simulink model "flo1_2018a"  (R2018a)
settings: Solver=FixedStepAuto  StartTime=0.0  StopTime=inf  FixedStep=0.01  RelTol=1e-3  EnableMultiTasking=on
settings Model: EnablePacing=on  Creator=Florian  LastModifiedBy=Florian
settings SolverCC: AutoInsertRateTranBlk=on
settings DataIOCC: LimitDataPoints=on  ReturnWorkspaceOutputs=on
settings OptimizationCC: LifeSpan=inf
settings DebuggingCC: AllowSymbolicDim=off  SFUnexpectedBacktrackingDiag=warning  SFNoUnconditionalDefaultTransitionDiag=warning  SFExecutionAtInitializationDiag=none  SFMachineParentedDataDiag=error
settings CodeAppCC: StateflowObjectComments=on
settings GRTTargetCC: TargetLangStandard=C89/C90 (ANSI)
settings ConfigComp: CovMetricSettings=dw  CovSaveCumulativeToWorkspaceVar=on  CovSaveSingleToWorkspaceVar=on  CovExternalEMLEnable=off  CovSFcnEnable=off

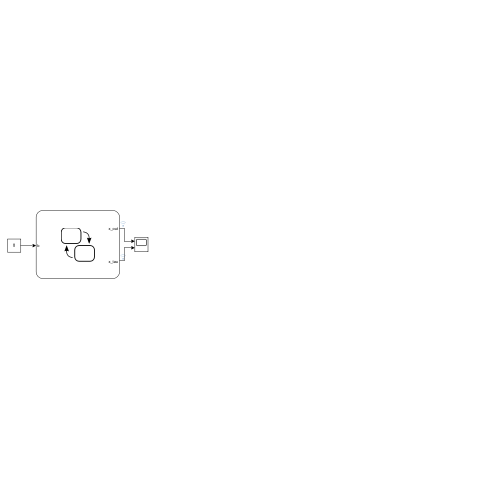
[thumbnail: Simulink's stored preview of the top-level diagram]
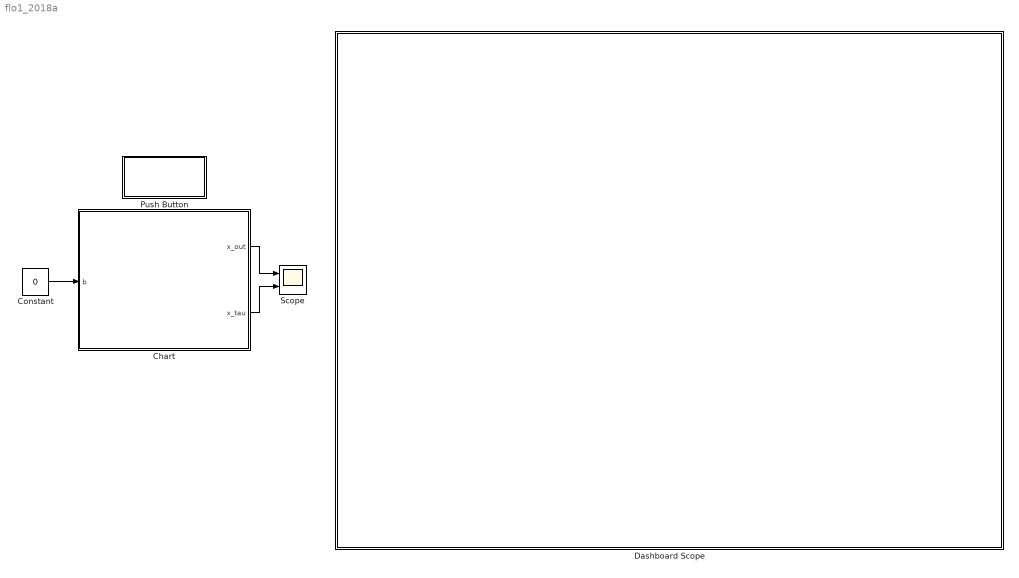
== system flo1_2018a ==
  Chart : Stateflow chart  TreatAsAtomicUnit=on
  Constant : Constant  Value=0
  Dashboard Scope : Subsystem  DialogController=hmiCreateDDGDialog  IsWebBlock=on  mask(MWDashboardBlock){webBlockId=8229a94b-91c7-4175-8aa9-2c0e1a5239d7, webBlockType=sdiscope, ShowInLibBrowser=on, ShowInitialText=on, HMISrcModelName=flo1_2018b}
      mask prompts: webBlockId "WebBlock Id"; webBlockType "WebBlock Type"; HMISrcModelName "Source Model"
      mask help: Traces signals on the dashboard scope during simulation.
      mask Help: helpview([docroot '/mapfiles/simulink.map'], 'hmi_scope')
      mask Display:
      | if strcmp(get_param(bdroot(gcb),'BlockDiagramType'),'library')
      |  image([(matlabroot) '/toolbox/simulink/hmi/icons/SDIScope.png'])
      | end
  Push Button : Subsystem  DialogController=hmiCreateDDGDialog  IsWebBlock=on  mask(MWDashboardBlock){webBlockId=e2df59ab-c7d6-43ec-aab9-14b79f501381, webBlockType=pushbutton, ShowInLibBrowser=on, ShowInitialText=on, HMISrcModelName=flo1_2018b}
      mask prompts: webBlockId "WebBlock Id"; webBlockType "WebBlock Type"; HMISrcModelName "Source Model"
      mask help: Change the value of a variable or tunable parameter using a button. You can configure the button to respond to a click by momentarily changing the value until you release or by latching the value until you click again.
      mask Help: helpview([docroot '/mapfiles/simulink.map'], 'hmi_pushbutton')
      mask Display:
      | if strcmp(get_param(bdroot(gcb),'BlockDiagramType'),'library')
      |  image([(matlabroot) '/toolbox/simulink/hmi/icons/PushButton.png'])
      | end
  Scope : Scope  NumInputPorts=2
  wires:
  Chart/1(x_out) -> Scope/1
  Chart/2(x_tau) -> Scope/2
  Constant/1 -> Chart/1(b)

== system flo1_2018a/Dashboard Scope ==

== system flo1_2018a/Push Button ==

== stateflow chart flo1_2018a/Chart ==
  settings: updateMethod=CONTINUOUS  executeAtInitialization=1  initializeOutput=1
  state Q0
    du:
    %derivative
    x_dot=0;
    tau_dot=0;
    %output
    x_out = x;
    x_tau = tau;
  state Q1
    du:
    %derivative
    x_dot=-alpha;
    tau_dot=1;
    %output
    x_out = x;
    x_tau = tau;
  (default) -> Q0 : {x =100
      | tau = 0}
  Q0 -> Q1 : [b]{tau = 0}
  Q1 -> Q0 : [tau >= tau_max]
  data: x local double; tau local double; x_out output double size=1; x_tau output double size=1; tau_max constant double =10; alpha constant double =3; b input
  data x settings: updateMethod=SF_CONTINUOUS_TIME_DATA
  data tau settings: updateMethod=SF_CONTINUOUS_TIME_DATA
